simulink model "qs2_ass"  (R2022b)
settings: Solver=VariableStepAuto  StartTime=0.0  StopTime=35  RelTol=1e-3
libraries: simulink_extras x1
settings Model: Creator=sohamkarak  LastModifiedBy=sohamkarak

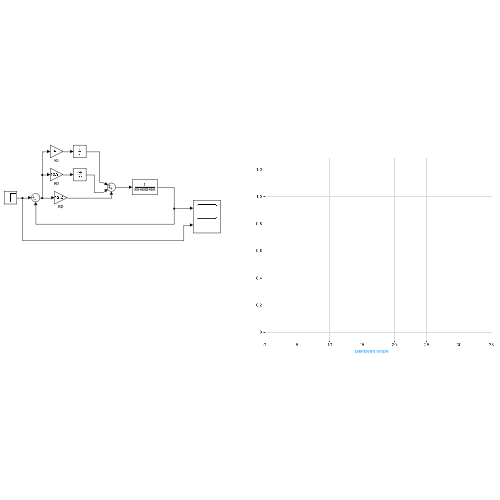
[thumbnail: Simulink's stored preview of the top-level diagram]
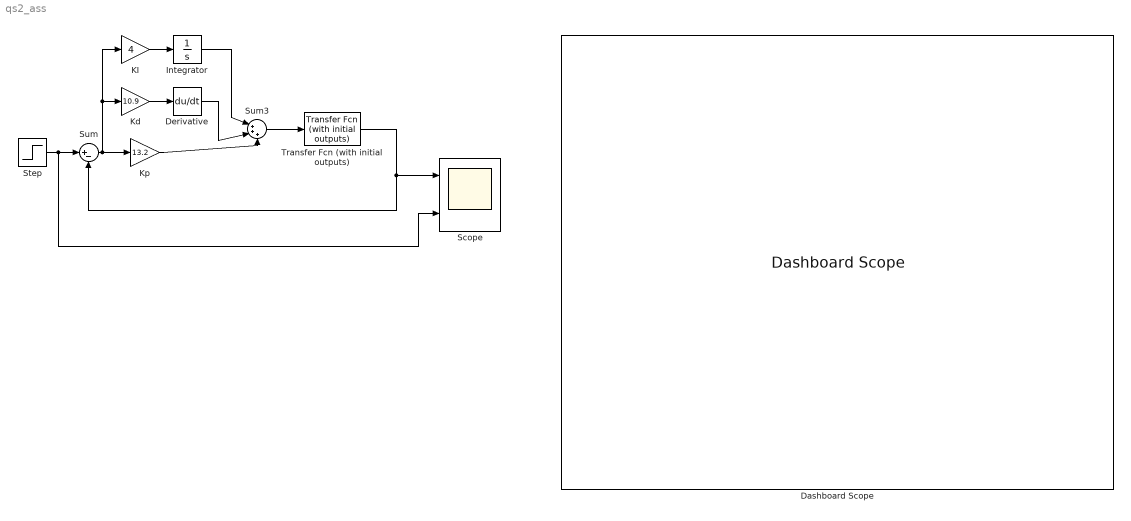
== system qs2_ass ==
  Dashboard Scope : DashboardScope
  Derivative : Derivative
  Integrator : Integrator
  KI : Gain  Gain=4
  Kd : Gain  Gain=10.9
  Kp : Gain  Gain=13.2
  Scope : Scope  NumInputPorts=2
  Step : Step  Time=0.1  SampleTime=0
  Sum : Sum  Inputs=|+-
  Sum3 : Sum  Inputs=|+++
  Transfer Fcn (with initial outputs) : simulink_extras/Additional Linear/Transfer Fcn (with initial outputs)  N=[1]  D=[1 6 5 0]  Y0=0  U0=0
  wires:
  Step/1 -> Scope/2, Sum/1
  Sum/1 -> Kd/1, KI/1, Kp/1
  Transfer Fcn (with initial outputs)/1 -> Sum/2, Scope/1
  Sum3/1 -> Transfer Fcn (with initial outputs)/1
  Kp/1 -> Sum3/3
  Kd/1 -> Derivative/1
  Integrator/1 -> Sum3/1
  Derivative/1 -> Sum3/2
  KI/1 -> Integrator/1
